simulink model "Cart_Pendulum_Linear"  (R2019b)
settings: Solver=VariableStepAuto  StartTime=0.0  StopTime=10.0  RelTol=1e-3
undefined symbols (not defined in the file or in its folder): A_mat, B_mat, C_mat, D_mat
settings Model: Creator=don  LastModifiedBy=don

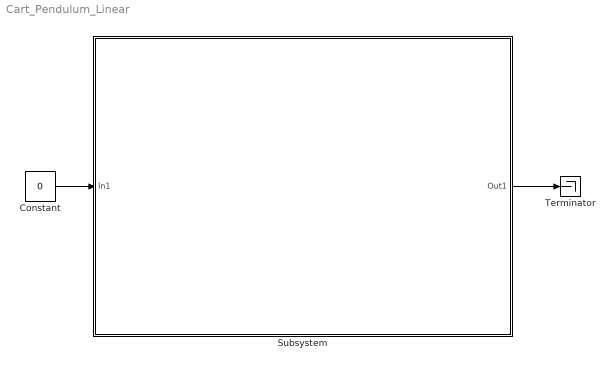
== system Cart_Pendulum_Linear ==
  Constant : Constant  Value=0
  Subsystem : Subsystem
  Terminator : Terminator
  wires:
  Constant/1 -> Subsystem/1(In1)
  Subsystem/1(Out1) -> Terminator/1

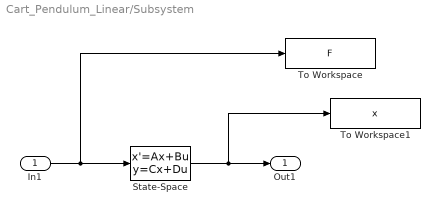
== system Cart_Pendulum_Linear/Subsystem ==
  In1 : Inport
  State-Space : StateSpace  A=A_mat  B=B_mat  C=C_mat  D=D_mat  InitialCondition=0
  To Workspace : ToWorkspace  VariableName=F  SaveFormat=Timeseries  SampleTime=-1
  To Workspace1 : ToWorkspace  VariableName=x  SaveFormat=Timeseries  SampleTime=-1
  Out1 : Outport
  wires:
  In1/1 -> To Workspace/1, State-Space/1
  State-Space/1 -> To Workspace1/1, Out1/1
